simulink model "model"  (R2018a)
settings: Solver=VariableStepAuto  StartTime=0.0  StopTime=70  RelTol=1e-3
settings Model: Creator=winfer  LastModifiedBy=winfer

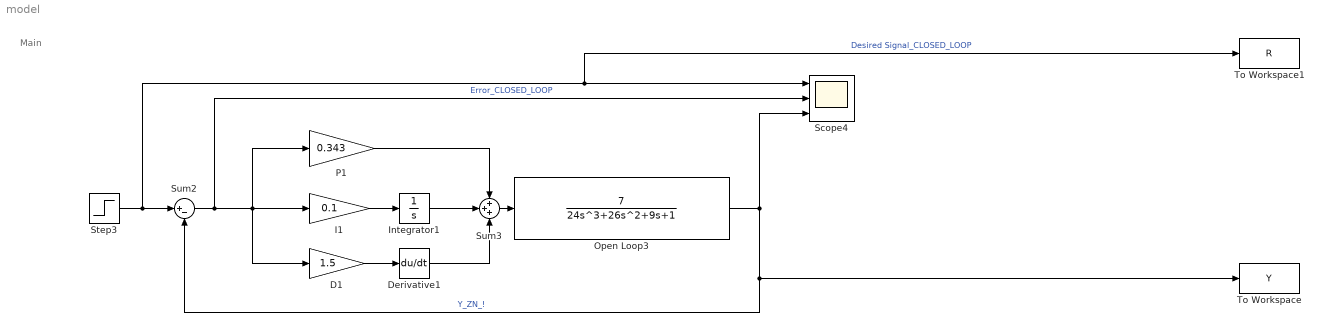
== system model ==
  note: Main
  D1 : Gain  Gain=1.5
  Derivative1 : Derivative
  I1 : Gain  Gain=0.1
  Integrator1 : Integrator
  Open Loop3 : TransferFcn  Numerator=[7]  Denominator=[24 26 9 1]
  P1 : Gain  Gain=0.343
  Scope4 : Scope  NumInputPorts=3
  Step3 : Step  Time=0  SampleTime=0
  Sum2 : Sum  Inputs=|+-
  Sum3 : Sum  Inputs=+++
  To Workspace : ToWorkspace  VariableName=Y  SaveFormat=Timeseries
      settings: Save2DSignal=2-D array (concatenate along first dimension)
  To Workspace1 : ToWorkspace  VariableName=R  SaveFormat=Timeseries
      settings: Save2DSignal=2-D array (concatenate along first dimension)
  wires:
  Open Loop3/1 -> To Workspace/1, Sum2/2, Scope4/3  "Y_ZN_!"
  Sum3/1 -> Open Loop3/1
  I1/1 -> Integrator1/1
  Integrator1/1 -> Sum3/2
  D1/1 -> Derivative1/1
  P1/1 -> Sum3/1
  Derivative1/1 -> Sum3/3
  Sum2/1 -> D1/1, P1/1, I1/1, Scope4/2  "Error_CLOSED_LOOP"
  Step3/1 -> Sum2/1, To Workspace1/1, Scope4/1  "Desired Signal_CLOSED_LOOP"
